simulink model "heli_azimut2_harness1"  (R2020b)
settings: Solver=daessc  StartTime=0.0  StopTime=50  MaxStep=1e-2  RelTol=1e-3  AbsTol=1e-4  EnableMultiTasking=on
libraries: simulink x1
settings Model: OrderedModelArguments=off  Creator=najman.jan  LastModifiedBy=artem
settings SolverCC: AutoScaleAbsTol=off
settings DataIOCC: LimitDataPoints=on  SaveOutput=off  SaveTime=off  SignalLoggingName=logsout_helicop
settings OptimizationCC: LifeSpan=inf
settings DebuggingCC: SolverPrmCheckMsg=warning  UnconnectedInputMsg=none  UnconnectedOutputMsg=none  AllowSymbolicDim=off  SFUnexpectedBacktrackingDiag=warning  SFNoUnconditionalDefaultTransitionDiag=warning  SFExecutionAtInitializationDiag=none  ArithmeticOperatorsInVariantConditions=warning
settings HardwareCC: ProdBitPerPointer=32  ProdBitPerSizeT=32  ProdBitPerPtrDiffT=32  ProdLargestAtomicFloat=None  ProdIntDivRoundTo=Undefined  ProdEndianess=Unspecified  ProdWordSize=32  ProdHWDeviceType=32-bit Generic
settings ModelReferenceCC: PropagateSignalLabelsOutOfModel=off
settings SFSimCC: SimUseLocalCustomCode=off  CustomCodeUndefinedFunction=UseInterfaceOnly
settings RTWCC: RTWUseLocalCustomCode=off
settings CodeAppCC: GenerateComments=off  StateflowObjectComments=on
settings GRTTargetCC: TargetLangStandard=C89/C90 (ANSI)
settings ConfigComp: CovMetricSettings=dw  CovSaveCumulativeToWorkspaceVar=on  CovSaveSingleToWorkspaceVar=on  CovExternalEMLEnable=off  CovSFcnEnable=off
settings SimscapeCC: SimscapeNormalizeSystem=off  SimscapeLogSimulationStatistics=on  SimscapeLogName=simlog_sm_single_pendulum_sl  SimscapeLogDataHistory=10000
settings ConfigurationSet: Description=SimMechanics 2G
settings ExplorerConfigSet: InternalSimMechanicsExplorerSettings="<ExplorerConfiguration><canonicalview>planar_xy</canonicalview><AnimationSetting><BasePlaybackSpeed>1.0</BasePlaybackSpeed><PlaybackSpeedFactor>1.0</PlaybackSpeedFactor></AnimationSetting><TilePanel><TileInfo><Tiles Columns=\"1\" Count=\"1\" Rows=\"1\"><Column Left=\"2\" Weight=\"1\"/><Column Left=\"750\"/><Row Top=\"2\" Weight=\"1\"/><Row Top=\"518\"/><Tile Height=\"1\" Width=\"1\" X=\"0\" Y=\"0\"/></Tiles></TileInfo><SceneInfo><SceneViewer><BGColor><R>0.60000002384185791</R><G>0.60000002384185791</G><B>0.60000002384185791</B></BGColor><Camera><Position><X>0.0048430711030960083</X><Y>-0.600354611873626709</Y><Z>2.1186925158267691</Z></Position><Center><X>0.0048430711030960083</X><Y>-0.600354611873626709</Y><Z>0</Z></Center><Up><X>0</X><Y>1</Y><Z>-0</Z></Up><Left>-0.110085226222872742</Left><Right>0.110085226222872742</Right><Bottom>-0.735372367501258895</Bottom><Top>0.735372367501258895</Top></Camera></SceneViewer></SceneInfo></TilePanel></ExplorerConfiguration>"

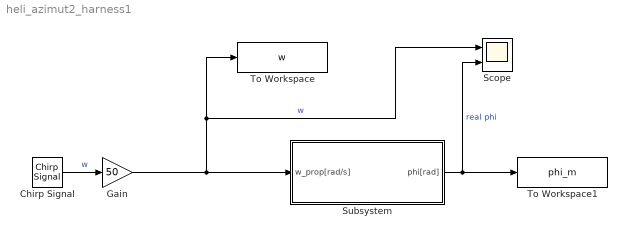
== system heli_azimut2_harness1 ==
  Chirp Signal : simulink/Sources/Chirp Signal  f1=0.1  T=100  f2=1
  Gain : Gain  Gain=50
  Scope : Scope  NumInputPorts=2
  Subsystem : Subsystem
  To Workspace : ToWorkspace  VariableName=w  SaveFormat=Timeseries  SampleTime=-1
  To Workspace1 : ToWorkspace  VariableName=phi_m  SaveFormat=Timeseries  SampleTime=-1
  wires:
  Subsystem/1(phi[rad]) -> To Workspace1/1, Scope/2  "real phi"
  Chirp Signal/1 -> Gain/1  "w"
  Gain/1 -> Scope/1, To Workspace/1, Subsystem/1(w_prop[rad/s])  "w"

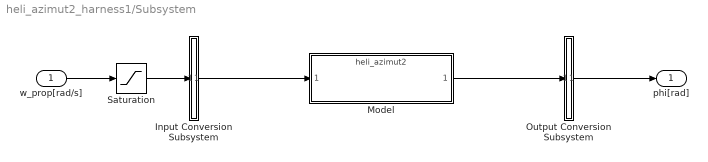
== system heli_azimut2_harness1/Subsystem ==
  w_prop[rad/s] : Inport  OutDataTypeStr=double  PortDimensions=[1]  SampleTime=0
  Input Conversion Subsystem : Subsystem  Tag=__SLT_ICS__  Description=|
      | Signal spec.
      | and routing
      settings: AttributesFormatString=%<Description>
  Model : ModelReference  ModelNameDialog=heli_azimut2.slxp  ModelReferenceVersion=1.106  CopyOfModelProtected=on
  Output Conversion Subsystem : Subsystem  Tag=__SLT_OCS__  Description=|
      | Signal spec.
      | and routing
      settings: AttributesFormatString=%<Description>
  Saturation : Saturate  UpperLimit=125  LowerLimit=-125
  phi[rad] : Outport
  wires:
  Model/1 -> Output Conversion Subsystem/1(Inport_1)
  Output Conversion Subsystem/1(Outport_1) -> phi[rad]/1
  Saturation/1 -> Input Conversion Subsystem/1(Inport_1)
  w_prop[rad/s]/1 -> Saturation/1
  Input Conversion Subsystem/1(Outport_1) -> Model/1

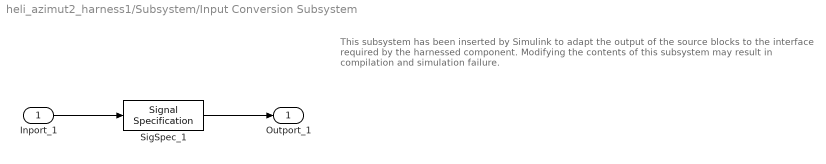
== system heli_azimut2_harness1/Subsystem/Input Conversion Subsystem ==
  note: This subsystem has been inserted by Simulink to adapt the output of the source blocks to the interface required by the harnessed component.
      |  Modifying the contents of this subsystem may result in compilation and simulation failure.
  Inport_1 : Inport
  SigSpec_1 : SignalSpecification  OutDataTypeStr=double  Dimensions=[1]  SampleTime=[0, 0]
  Outport_1 : Outport
  wires:
  SigSpec_1/1 -> Outport_1/1
  Inport_1/1 -> SigSpec_1/1

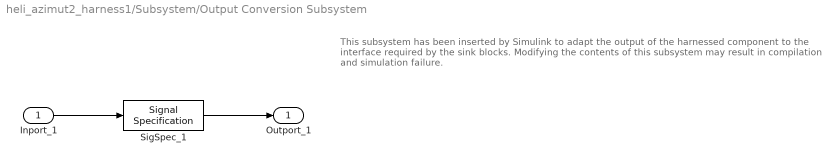
== system heli_azimut2_harness1/Subsystem/Output Conversion Subsystem ==
  note: This subsystem has been inserted by Simulink to adapt the output of the harnessed component to the interface required by the sink blocks.
      |  Modifying the contents of this subsystem may result in compilation and simulation failure.
  Inport_1 : Inport
  SigSpec_1 : SignalSpecification  OutDataTypeStr=double  Unit=rad  Dimensions=[1]
  Outport_1 : Outport
  wires:
  Inport_1/1 -> SigSpec_1/1
  SigSpec_1/1 -> Outport_1/1
